simulink model "modelorecuperadorclock6_4"  (Simulink 7.5)
settings: Solver=ode45  StartTime=0.0  StopTime=10.0  RelTol=1e-3
libraries: simulink x2, commsynccomp2 x1, dspsigops x1, simulink_extras x1
settings Model: Creator=Francisco  LastModifiedBy=Francisco

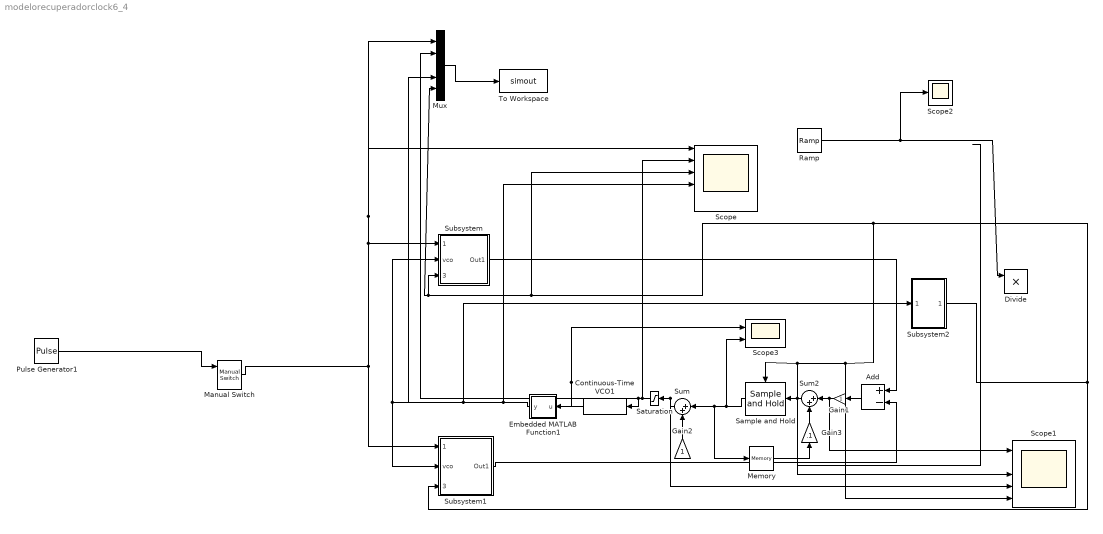
== system modelorecuperadorclock6_4 ==
  Add : Sum  Inputs=+-  OutDataType=fixdt(1, 16)  OutScaling=2^-10
  Continuous-Time VCO1 : commsynccomp2/Continuous-Time VCO  SystemSampleTime=-1  Ac=1  Fc=1  Kc=0.5  Ph=pi/2
  Divide : Product  Inputs=**  OutDataType=fixdt(1, 16)  OutScaling=2^-10
  Embedded MATLAB Function1 : Stateflow chart  TreatAsAtomicUnit=on
  Gain1 : Gain  ParameterDataType=fixdt(1, 16)  ParameterScaling=2^0  OutDataType=fixdt(1, 16)  OutScaling=2^0
  Gain2 : Gain  ParameterDataType=fixdt(1, 16)  ParameterScaling=2^0  OutDataType=fixdt(1, 16)  OutScaling=2^0
  Gain3 : Gain  Gain=.1  ParameterDataType=fixdt(1, 16)  ParameterScaling=2^0  OutDataType=fixdt(1, 16)  OutScaling=2^0
  Manual Switch : simulink/Signal Routing/Manual Switch  SystemSampleTime=-1  sw=1  action=0  varsize=off
  Memory : Memory
  Mux : Mux  Inputs=5
  Pulse Generator1 : DiscretePulseGenerator  PulseType=Time based  Amplitude=1  Period=2.2  PulseWidth=50  PhaseDelay=0  SampleTime=1
  Ramp : simulink/Sources/Ramp  SystemSampleTime=-1  slope=0.4/200  start=0  X0=0.1
  Sample and Hold : dspsigops/Sample and Hold  SystemSampleTime=-1  trig=Falling edge  initCond=0  latchinput=off
  Saturation : Saturate  UpperLimit=10  LowerLimit=-10  OutDataType=fixdt(1, 16)  OutScaling=2^0
  Scope : Scope  NumInputPorts=6
      settings: YMin=-1~-5~-5~-5~-5~-1  YMax=2~5~5~5~5~2
  Scope1 : Scope  NumInputPorts=5
      settings: YMin=-0.15~-0.0605~-0.2~-0.189~-5  YMax=0.45~-0.0555~0.4~-0.174~5  SaveName=ScopeData4
  Scope2 : Scope
      settings: SaveName=ScopeData5
  Scope3 : Scope  NumInputPorts=2
      settings: TimeRange=200  YMin=-1~-5  YMax=1~5  SaveName=ScopeData3
  Subsystem : Subsystem
  Subsystem1 : Subsystem
  Subsystem2 : Subsystem
  Sum : Sum  Inputs=|++  OutDataType=fixdt(1, 16)  OutScaling=2^0
  Sum2 : Sum  Inputs=|++  OutDataType=fixdt(1, 16)  OutScaling=2^0
  To Workspace : ToWorkspace  VariableName=simout  SampleTime=-1  SaveFormat=Structure With Time
  wires:
  Subsystem1/1(Out1) -> Add/2
  Subsystem/1(Out1) -> Add/1
  Subsystem2/1(Out1) -> Subsystem/3(div frecuensia), Mux/5, Scope/3, Sample and Hold/Trigger, Scope1/5, Subsystem1/3(div frecuensia)
  Sample and Hold/1 -> Scope3/2, Sum/1, Memory/1
  Continuous-Time VCO1/1 -> Scope3/1, Embedded MATLAB Function1/1(u)
  Manual Switch/1 -> Subsystem1/1(señal original), Subsystem/1(señal orginal), Mux/1, Scope/1
  Embedded MATLAB Function1/1(y) -> Subsystem/2(vco), Subsystem1/2(vco), Subsystem2/1(In1), Mux/4, Scope/4
  Mux/1 -> To Workspace/1
  Pulse Generator1/1 -> Manual Switch/1
  Sum/1 -> Saturation/1, Scope1/4
  Saturation/1 -> Mux/2, Continuous-Time VCO1/1, Scope/2
  Sum2/1 -> Sample and Hold/1, Scope1/3
  Add/1 -> Gain1/1
  Gain1/1 -> Sum2/1, Scope1/1
  Gain2/1 -> Sum/2
  Ramp/1 -> Divide/1, Scope2/1
  Gain3/1 -> Sum2/2
  Memory/1 -> Gain3/1

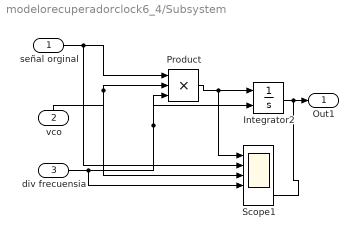
== system modelorecuperadorclock6_4/Subsystem ==
  señal orginal : Inport
  vco : Inport  Port=2
  div frecuensia : Inport  Port=3
  Integrator2 : Integrator  ExternalReset=rising
  Product : Product  Inputs=3  OutDataType=fixdt(1, 16)  OutScaling=2^0  RndMeth=Zero
  Scope1 : Scope  NumInputPorts=5
      settings: YMin=-5~-5~-5~-5~-5  YMax=5~5~5~5~5
  Out1 : Outport
  wires:
  div frecuensia/1 -> Scope1/4, Integrator2/2, Product/3
  Product/1 -> Integrator2/1, Scope1/1
  señal orginal/1 -> Scope1/2, Product/1
  vco/1 -> Scope1/3, Product/2
  Integrator2/1 -> Out1/1, Scope1/5

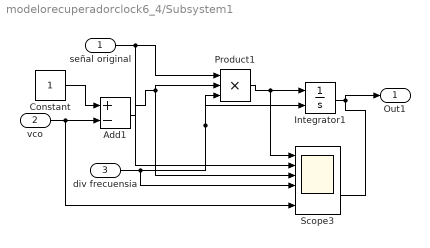
== system modelorecuperadorclock6_4/Subsystem1 ==
  señal original : Inport
  vco : Inport  Port=2
  div frecuensia : Inport  Port=3
  Add1 : Sum  Inputs=+-  OutDataType=fixdt(1, 16)  OutScaling=2^-10
  Constant : Constant  OutDataType=fixdt(1, 16)  OutScaling=2^0
  Integrator1 : Integrator  ExternalReset=rising
  Product1 : Product  Inputs=3  OutDataType=fixdt(1, 16)  OutScaling=2^0  RndMeth=Zero
  Scope3 : Scope  NumInputPorts=6
      settings: YMin=-5~-5~-5~-5~-5~-5  YMax=5~5~5~5~5~5  SaveName=ScopeData2
  Out1 : Outport
  wires:
  Product1/1 -> Integrator1/1, Scope3/1
  señal original/1 -> Scope3/2, Product1/1
  Add1/1 -> Product1/2, Scope3/3
  div frecuensia/1 -> Scope3/4, Integrator1/2, Product1/3
  Constant/1 -> Add1/1
  Integrator1/1 -> Out1/1, Scope3/5
  vco/1 -> Add1/2, Scope3/6

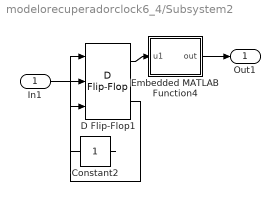
== system modelorecuperadorclock6_4/Subsystem2 ==
  In1 : Inport
  Constant2 : Constant  OutDataType=fixdt(1, 16)  OutScaling=2^0
  D Flip-Flop1 : simulink_extras/Flip Flops/D Flip-Flop  SystemSampleTime=-1
  Embedded MATLAB Function4 : Stateflow chart  TreatAsAtomicUnit=on
  Out1 : Outport
  wires:
  D Flip-Flop1/2 -> D Flip-Flop1/1
  Constant2/1 -> D Flip-Flop1/3
  In1/1 -> D Flip-Flop1/2
  D Flip-Flop1/1 -> Embedded MATLAB Function4/1(u1)
  Embedded MATLAB Function4/1(out) -> Out1/1

== matlab function Embedded MATLAB Function1 ==
  data: u input double; y output double
function y = diferenciador(u)
%#eml
ref=0;
k=0;
if u>=ref
    k=1;
end
if u<ref
    k=0;
end
 y=k;
end

== matlab function Subsystem2/Embedded MATLAB Function4 ==
  data: u1 input double; out output double
function out  = inv(u1)
out=1-u1;
end
